simulink model "fig7_46"  (Simulink 7.9)
settings: Solver=ode45  StartTime=0.0  StopTime=5  RelTol=1e-3
settings Model: Creator=abbas  LastModifiedBy=abbas  ExtModeTrigMode=oneshot  ExtModeArmWhenConnect=off
settings DataIOCC: LimitDataPoints=off
settings OptimizationCC: BlockReduction=off  BooleanDataType=off  InlineInvariantSignals=on  InitFltsAndDblsToZero=on
settings DebuggingCC: SaveWithParameterizedLinksMsg=none  SignalResolutionControl=TryResolveAllWithWarning  SolverPrmCheckMsg=none  MultiTaskDSMMsg=warning  MultiTaskCondExecSysMsg=none  FcnCallInpInsideContextMsg=Use local settings  StrictBusMsg=None
settings HardwareCC: TargetUnknown=on
settings RTWCC: IncludeERTFirstTime=on
settings GRTTargetCC: TargetFcnLib=ansi_tfl_tmw.mat  ModelReferenceCompliant=off  ParMdlRefBuildCompliant=off  CompOptLevelCompliant=off  ConcurrentExecutionCompliant=off  CombineOutputUpdateFcns=off  MatFileLogging=off  GRTInterface=on

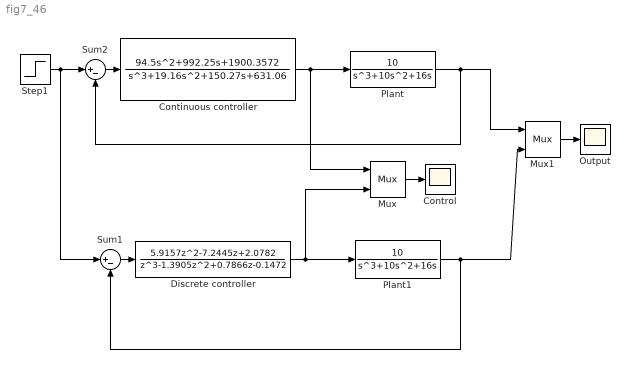
== system fig7_46 ==
  Continuous controller : TransferFcn  Numerator=[94.5 992.25 1900.3572]  Denominator="[1 19.16  150.27 631.06]"
  Control : Scope
      settings: TickLabels=on  YMin=0  YMax=2.75  SaveName=ucd
  Discrete controller : DiscreteTransferFcn  Numerator=[5.9157 -7.2445 2.0782]  Denominator=[1 -1.3905 0.7866 -0.1472]  SampleTime=.1
  Mux : Mux  Inputs=2
  Mux1 : Mux  Inputs=2
  Output : Scope
      settings: TickLabels=on  SaveName=ycd
  Plant : TransferFcn  Numerator=[10]  Denominator="[1  10 16 0]"
  Plant1 : TransferFcn  Numerator=[10]  Denominator="[1  10 16 0]"
  Step1 : Step  Time=0  SampleTime=.01
  Sum1 : Sum  Inputs=|+-  InputSameDT=on  OutDataTypeStr=Inherit: Same as first input
  Sum2 : Sum  Inputs=|+-  InputSameDT=on  OutDataTypeStr=Inherit: Same as first input
  wires:
  Mux/1 -> Control/1
  Mux1/1 -> Output/1
  Sum1/1 -> Discrete controller/1
  Plant/1 -> Mux1/1, Sum2/2
  Sum2/1 -> Continuous controller/1
  Continuous controller/1 -> Plant/1, Mux/1
  Discrete controller/1 -> Plant1/1, Mux/2
  Plant1/1 -> Sum1/2, Mux1/2
  Step1/1 -> Sum2/1, Sum1/1
